simulink subsystem "VCM_main"  (R2021b)
settings: Solver=VariableStepAuto  StartTime=0.0  StopTime=10.0  RelTol=1e-3
values from neighbouring files (symbols this model uses):
  g = 9.80665    [VehicleParamsFEM20_Gear17.m]
  gear_f = 14.45    [VehicleParamsFEM20_Gear17.m]
  gear_r = 14.45    [VehicleParamsFEM20_Gear17.m]
  Iwf = 0.2    [VehicleParamsFEM20_Gear17.m]
  Rwf = 18*(25.4/1000)/2    (= 0.2286)    [VehicleParamsFEM20_Gear17.m]
libraries: simulink x46, dspswit3 x1, slpidlib x1
(part 5 of 5)

== system VCM_main/VDC/VCM_Status/Sliprate/Sliprate Calculator ==
  <VELOCITY_X> : Inport
  <MC4_Actual speed value in 1/rpm> : Inport  Port=2
  <MC2_Actual speed value in 1/rpm> : Inport  Port=3
  <MC3_Actual speed value in 1/rpm> : Inport  Port=4
  <MC1_Actual speed value in 1/rpm> : Inport  Port=5
  FL_Sliprate Caluclator : Subsystem
  FR_Sliprate Caluclator : Subsystem
  RL_Sliprate Caluclator : Subsystem
  RR_Sliprate Caluclator : Subsystem
  FL_Sliprate : Outport
  RR_Sliprate : Outport  Port=2
  RL_Sliprate : Outport  Port=3
  FR_Sliprate : Outport  Port=4
  wires:
  RL_Sliprate Caluclator/1(RL_Sliprate) -> RL_Sliprate/1
  RR_Sliprate Caluclator/1(RR_Sliprate) -> RR_Sliprate/1
  FL_Sliprate Caluclator/1(FL_Sliprate) -> FL_Sliprate/1
  <MC4_Actual speed value in 1/rpm>/1 -> FL_Sliprate Caluclator/2(<MC4_Actual speed value in 1/rpm>)
  <VELOCITY_X>/1 -> FL_Sliprate Caluclator/1(<VELOCITY_X>), RR_Sliprate Caluclator/1(<VELOCITY_X>), FR_Sliprate Caluclator/1(<VELOCITY_X>), RL_Sliprate Caluclator/1(<VELOCITY_X>)
  <MC2_Actual speed value in 1/rpm>/1 -> RR_Sliprate Caluclator/2(<MC2_Actual speed value in 1/rpm>)
  <MC3_Actual speed value in 1/rpm>/1 -> RL_Sliprate Caluclator/2(<MC3_Actual speed value in 1/rpm>)
  FR_Sliprate Caluclator/1(FR_Sliprate) -> FR_Sliprate/1
  <MC1_Actual speed value in 1/rpm>/1 -> FR_Sliprate Caluclator/2(<MC1_Actual speed value in 1/rpm>)

== system VCM_main/VDC/VCM_Status/Sliprate/Sliprate Calculator/FL_Sliprate Caluclator ==
  <VELOCITY_X> : Inport
  <MC4_Actual speed value in 1/rpm> : Inport  Port=2
  Add : Sum  Inputs=-+
  Avoid division by zero : Subsystem
  Divide : Product  Inputs=*/
  Gear : Gain  Gain=13.75
  toTire_rpm : Gain  Gain=60/(2*pi*0.228)
  FL_Sliprate : Outport
  wires:
  Avoid division by zero/1(Out1) -> Divide/2
  Add/1 -> Divide/1
  <VELOCITY_X>/1 -> toTire_rpm/1
  Divide/1 -> FL_Sliprate/1  "FL_Sliprate"
  Gear/1 -> Add/1
  toTire_rpm/1 -> Gear/1
  <MC4_Actual speed value in 1/rpm>/1 -> Add/2, Avoid division by zero/1(In1)

== system VCM_main/VDC/VCM_Status/Sliprate/Sliprate Calculator/FR_Sliprate Caluclator ==
  <VELOCITY_X> : Inport
  <MC1_Actual speed value in 1/rpm> : Inport  Port=2
  Add : Sum  Inputs=-+
  Avoid division by zero : Subsystem
  Divide : Product  Inputs=*/
  Gear : Gain  Gain=13.75
  toTire_rpm : Gain  Gain=60/(2*pi*0.228)
  FR_Sliprate : Outport
  wires:
  Avoid division by zero/1(Out1) -> Divide/2
  Add/1 -> Divide/1
  <VELOCITY_X>/1 -> toTire_rpm/1
  Divide/1 -> FR_Sliprate/1  "FR_Sliprate"
  Gear/1 -> Add/1
  toTire_rpm/1 -> Gear/1
  <MC1_Actual speed value in 1/rpm>/1 -> Avoid division by zero/1(<MC1_Actual speed value in 1/rpm>), Add/2

== system VCM_main/VDC/VCM_Status/Sliprate/Sliprate Calculator/RL_Sliprate Caluclator ==
  <VELOCITY_X> : Inport
  <MC3_Actual speed value in 1/rpm> : Inport  Port=2
  Add : Sum  Inputs=-+
  Avoid division by zero : Subsystem
  Divide : Product  Inputs=*/
  Gear : Gain  Gain=13.75
  toTire_rpm : Gain  Gain=60/(2*pi*0.228)
  RL_Sliprate : Outport
  wires:
  Avoid division by zero/1(Out1) -> Divide/2
  Add/1 -> Divide/1
  <VELOCITY_X>/1 -> toTire_rpm/1
  Divide/1 -> RL_Sliprate/1  "RL_Sliprate"
  Gear/1 -> Add/1
  toTire_rpm/1 -> Gear/1
  <MC3_Actual speed value in 1/rpm>/1 -> Avoid division by zero/1(<MC3_Actual speed value in 1/rpm>), Add/2

== system VCM_main/VDC/VCM_Status/Sliprate/Sliprate Calculator/RR_Sliprate Caluclator ==
  <VELOCITY_X> : Inport
  <MC2_Actual speed value in 1/rpm> : Inport  Port=2
  Add : Sum  Inputs=-+
  Avoid division by zero : Subsystem
  Divide : Product  Inputs=*/
  Gear : Gain  Gain=13.75
  toTire_rpm : Gain  Gain=60/(2*pi*0.228)
  RR_Sliprate : Outport
  wires:
  Avoid division by zero/1(Out1) -> Divide/2
  Add/1 -> Divide/1
  <VELOCITY_X>/1 -> toTire_rpm/1
  Divide/1 -> RR_Sliprate/1  "RR_Sliprate"
  Gear/1 -> Add/1
  toTire_rpm/1 -> Gear/1
  <MC2_Actual speed value in 1/rpm>/1 -> Avoid division by zero/1(<MC2_Actual speed value in 1/rpm>), Add/2

== system VCM_main/VDC/VCM_Status/Sliprate/Sliprate Calculator/FL_Sliprate Caluclator/Avoid division by zero ==
  In1 : Inport
  Compare To Zero : simulink/Logic and Bit Operations/Compare To Zero  relop===  OutDataTypeStr=boolean
  Constant : Constant  Value=eps
  Switch : Switch  Criteria=u2 > Threshold
  Out1 : Outport
  wires:
  Constant/1 -> Switch/1
  In1/1 -> Compare To Zero/1, Switch/3
  Compare To Zero/1 -> Switch/2
  Switch/1 -> Out1/1

== system VCM_main/VDC/VCM_Status/Sliprate/Sliprate Calculator/FR_Sliprate Caluclator/Avoid division by zero ==
  <MC1_Actual speed value in 1/rpm> : Inport
  Compare To Zero : simulink/Logic and Bit Operations/Compare To Zero  relop===  OutDataTypeStr=boolean
  Constant : Constant  Value=eps
  Switch : Switch  Criteria=u2 > Threshold
  Out1 : Outport
  wires:
  Constant/1 -> Switch/1
  <MC1_Actual speed value in 1/rpm>/1 -> Compare To Zero/1, Switch/3
  Compare To Zero/1 -> Switch/2
  Switch/1 -> Out1/1

== system VCM_main/VDC/VCM_Status/Sliprate/Sliprate Calculator/RL_Sliprate Caluclator/Avoid division by zero ==
  <MC3_Actual speed value in 1/rpm> : Inport
  Compare To Zero : simulink/Logic and Bit Operations/Compare To Zero  relop===  OutDataTypeStr=boolean
  Constant : Constant  Value=eps
  Switch : Switch  Criteria=u2 > Threshold
  Out1 : Outport
  wires:
  Constant/1 -> Switch/1
  <MC3_Actual speed value in 1/rpm>/1 -> Compare To Zero/1, Switch/3
  Compare To Zero/1 -> Switch/2
  Switch/1 -> Out1/1

== system VCM_main/VDC/VCM_Status/Sliprate/Sliprate Calculator/RR_Sliprate Caluclator/Avoid division by zero ==
  <MC2_Actual speed value in 1/rpm> : Inport
  Compare To Zero : simulink/Logic and Bit Operations/Compare To Zero  relop===  OutDataTypeStr=boolean
  Constant : Constant  Value=eps
  Switch : Switch  Criteria=u2 > Threshold
  Out1 : Outport
  wires:
  Constant/1 -> Switch/1
  <MC2_Actual speed value in 1/rpm>/1 -> Compare To Zero/1, Switch/3
  Compare To Zero/1 -> Switch/2
  Switch/1 -> Out1/1

== stateflow chart VCM_main/VDC/Launch/Chart ==
  state Base
    entry:
    LaunchTorqueLimit = MaxTorqueLimit;
    LaunchLED = 0;
  state OFF
    entry:
    LaunchTorqueLimit = 0;
  state LaunchReady
    entry:
    LaunchTorqueLimit = MaxTorqueLimit;
  state LaunchReady_BrakeON
    entry:
    LaunchTorqueLimit = 0;
    LaunchLED = 1;
  state LaunchReady_BrakeOff
    entry:
    LaunchTorqueLimit = 0;
    state LaunchLEDon
      entry:
      LaunchLED = 1;
    state LaunchLEDoff
      entry:
      LaunchLED = 0;
    (default) -> LaunchLEDon
    LaunchLEDoff -> LaunchLEDon : after(0.2,sec)
    LaunchLEDon -> LaunchLEDoff : after(0.2,sec)
  state LaunchGearProtection
    entry:
    LaunchTorqueLimit = GearProtectionTorqueLimit;
    LaunchLED = 1;
  (default) -> Base
  OFF -> Base : [Torque< 0.5]
  LaunchGearProtection -> Base : after(GearProtectionTime,sec)
  (junction 24) -> OFF
  Base -> LaunchReady : [LaunchSW == 1 & BrakeSW == 1 & rpm < 10 & Torque < 0.3]
  LaunchReady -> (junction 24) [order 2] : [LaunchSW == 0]
  (junction 17) -> (junction 24)
  LaunchReady -> LaunchReady_BrakeON [order 1] : after(2,sec)[BrakeSW == 1]
  LaunchReady_BrakeON -> (junction 17) [order 1] : [LaunchSW == 0]
  LaunchReady_BrakeON -> LaunchReady_BrakeOff [order 2] : after(1,sec)[BrakeSW == 0 & Torque > 5 ]
  LaunchReady_BrakeOff -> LaunchReady_BrakeON [order 1] : [Torque < 4 | BrakeSW == 1]
  LaunchReady_BrakeOff -> LaunchGearProtection [order 2] : [LaunchSW == 0]
  data: LaunchSW input; BrakeSW input; rpm input; Torque input; MaxTorqueLimit input; GearProtectionTorqueLimit input; GearProtectionTime input; LaunchLED output; LaunchTorqueLimit output
